simulink model "combinedTxRx"  (R2018a)
settings: Solver=FixedStepDiscrete  StartTime=0.0  StopTime=10.0  RelTol=1e-3
InitFcn:
  | modelSettings
values from neighbouring files (symbols this model uses):
  RadioSampleRate = 1e6    (= 1000000)    [modelSettings.m]
libraries: RxTxFixedPointLibrary x2, dspsigops x2, commsource2 x1
settings Model: Creator=tcollins  LastModifiedBy=fpgaws
settings OptimizationCC: BlockReduction=off  ConditionallyExecuteInputs=off  DefaultParameterBehavior=Inlined
settings DebuggingCC: AlgebraicLoopMsg=error  SingleTaskRateTransMsg=error  ParameterPrecisionLossMsg=none
settings HardwareCC: ProdBitPerPointer=32  ProdBitPerSizeT=32  ProdBitPerPtrDiffT=32  ProdLargestAtomicFloat=None  ProdIntDivRoundTo=Undefined  ProdEndianess=Unspecified  ProdWordSize=32  ProdHWDeviceType=ASIC/FPGA->ASIC/FPGA  ProdEqTarget=off
settings CodeAppCC: StateflowObjectComments=on

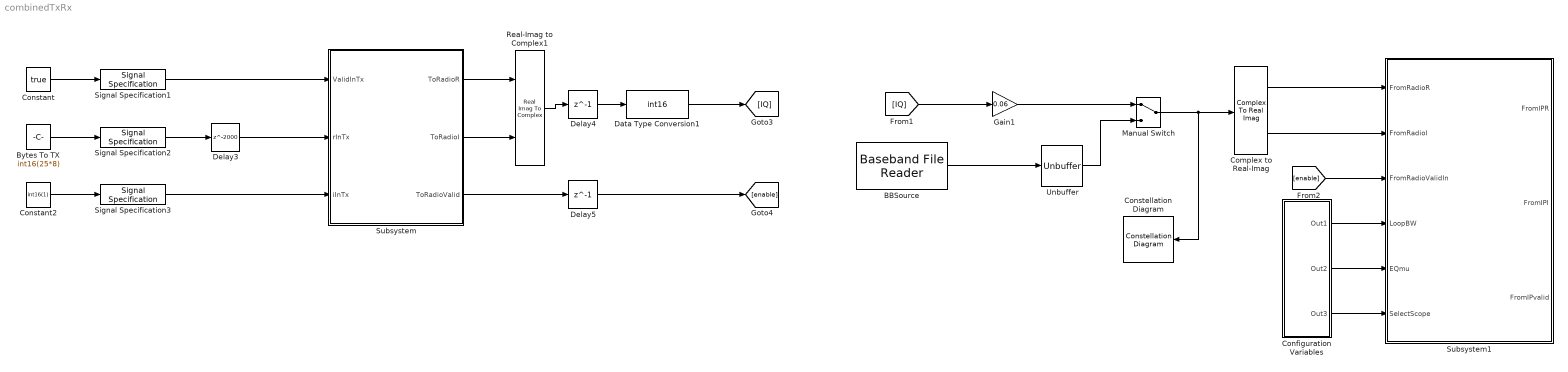
== system combinedTxRx ==
  BBSource : commsource2/Baseband File Reader  Filename=PlutoCaptureQPSK.bb  InheritSampleTimeFromFile=off  SampleTime=100000/(RadioSampleRate)  SamplesPerFrame=100000  CyclicRepetition=off  FileEndOutputPort=off  SimulateUsing=Interpreted execution
      settings: SourceProductName=Communications System Toolbox  SourceProductBaseCode=CM
  Bytes To TX : Constant  Value=int16(25*8)  SampleTime=-1
  Complex to Real-Imag : ComplexToRealImag
  Configuration Variables : Subsystem
  Constant : Constant  Value=true  SampleTime=-1
  Constant2 : Constant  Value=int16(1)  SampleTime=-1
  Constellation Diagram : ConstellationDiagram
  Data Type Conversion1 : DataTypeConversion  OutDataTypeStr=int16  ConvertRealWorld=Stored Integer (SI)
  Delay3 : Delay  DelayLength=2000
  Delay4 : Delay  DelayLength=1
  Delay5 : Delay  DelayLength=1
  Gain1 : Gain  Gain=0.06  OutDataTypeStr=int16
  Manual Switch : ManualSwitch
  Real-Imag to Complex1 : RealImagToComplex
  Signal Specification1 : SignalSpecification  OutDataTypeStr=boolean  SampleTime=1/RadioSampleRate
  Signal Specification2 : SignalSpecification  OutDataTypeStr=int16  SampleTime=1/RadioSampleRate
  Signal Specification3 : SignalSpecification  OutDataTypeStr=int16  SampleTime=1/RadioSampleRate
  Subsystem : Subsystem
  Subsystem1 : Subsystem
  Unbuffer : Unbuffer
  wires:
  Bytes To TX/1 -> Signal Specification2/1
  Constant2/1 -> Signal Specification3/1
  Constant/1 -> Signal Specification1/1
  BBSource/1 -> Unbuffer/1
  Signal Specification2/1 -> Delay3/1
  [IQ] -> Gain1/1
  Gain1/1 -> Manual Switch/1
  Unbuffer/1 -> Manual Switch/2
  Signal Specification1/1 -> Subsystem/1(ValidInTx)
  Delay3/1 -> Subsystem/2(rInTx)
  Signal Specification3/1 -> Subsystem/3(iInTx)
  Real-Imag to Complex1/1 -> Delay4/1
  Delay5/1 -> [enable]
  Data Type Conversion1/1 -> [IQ]
  Delay4/1 -> Data Type Conversion1/1
  Subsystem/3(ToRadioValid) -> Delay5/1
  Subsystem/1(ToRadioR) -> Real-Imag to Complex1/1
  Subsystem/2(ToRadioI) -> Real-Imag to Complex1/2
  Configuration Variables/1(Out1) -> Subsystem1/4(LoopBW)
  Configuration Variables/2(Out2) -> Subsystem1/5(EQmu)
  Configuration Variables/3(Out3) -> Subsystem1/6(SelectScope)
  [enable] -> Subsystem1/3(FromRadioValidIn)
  Complex to Real-Imag/2 -> Subsystem1/2(FromRadioI)
  Complex to Real-Imag/1 -> Subsystem1/1(FromRadioR)
  Manual Switch/1 -> Constellation Diagram/1, Complex to Real-Imag/1

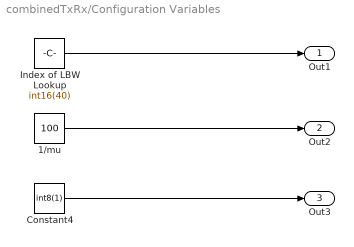
== system combinedTxRx/Configuration Variables ==
  1/mu : Constant  Value=100  OutDataTypeStr=int16  SampleTime=-1
  Constant4 : Constant  Value=int8(1)  SampleTime=1/RadioSampleRate
  Index of LBW Lookup : Constant  Value=int16(40)  SampleTime=1/RadioSampleRate
  Out1 : Outport
  Out2 : Outport  Port=2
  Out3 : Outport  Port=3
  wires:
  1/mu/1 -> Out2/1
  Index of LBW Lookup/1 -> Out1/1
  Constant4/1 -> Out3/1

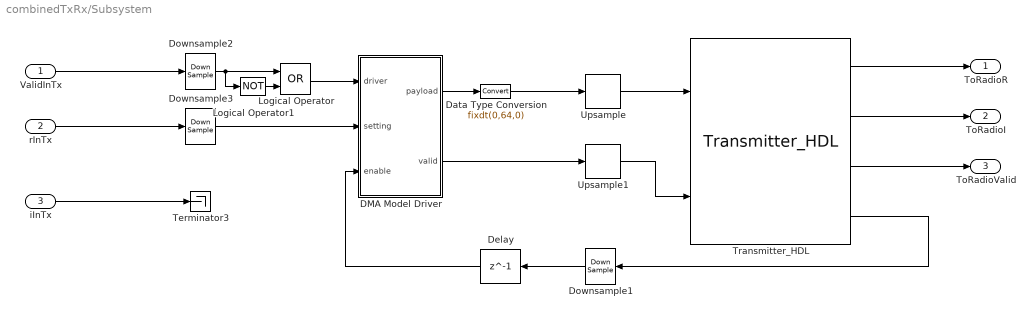
== system combinedTxRx/Subsystem ==
  ValidInTx : Inport
  rInTx : Inport  Port=2
  iInTx : Inport  Port=3
  DMA Model Driver : MATLAB Function  TreatAsAtomicUnit=on
  Data Type Conversion : DataTypeConversion  OutDataTypeStr=fixdt(0,64,0)
  Delay : Delay  DelayLength=1
  Downsample1 : DownSample  N=4  RateOptions=Allow multirate processing
  Downsample2 : DownSample  N=4  RateOptions=Allow multirate processing
  Downsample3 : DownSample  N=4  RateOptions=Allow multirate processing
  Logical Operator : Logic  Operator=OR  AllPortsSameDT=off  OutDataTypeStr=boolean
  Logical Operator1 : Logic  Operator=NOT  AllPortsSameDT=off  OutDataTypeStr=boolean
  Terminator3 : Terminator
  Transmitter_HDL : RxTxFixedPointLibrary/Transmitter_HDL  SystemSampleTime=-1
  Upsample : dspsigops/Upsample  N=4  phase=0  RateOptions=Allow multirate processing  ic=0  mode=Unused parameter value
  Upsample1 : dspsigops/Upsample  N=4  phase=0  RateOptions=Allow multirate processing  ic=0  mode=Unused parameter value
  ToRadioR : Outport
  ToRadioI : Outport  Port=2
  ToRadioValid : Outport  Port=3
  wires:
  Upsample/1 -> Transmitter_HDL/1
  Upsample1/1 -> Transmitter_HDL/2
  Transmitter_HDL/2 -> ToRadioI/1
  Downsample3/1 -> DMA Model Driver/2(setting)
  Logical Operator/1 -> DMA Model Driver/1(driver)
  Downsample2/1 -> Logical Operator/1, Logical Operator1/1
  iInTx/1 -> Terminator3/1
  Transmitter_HDL/4 -> Downsample1/1
  rInTx/1 -> Downsample3/1
  Data Type Conversion/1 -> Upsample/1
  DMA Model Driver/2(valid) -> Upsample1/1
  Transmitter_HDL/3 -> ToRadioValid/1
  Logical Operator1/1 -> Logical Operator/2
  DMA Model Driver/1(payload) -> Data Type Conversion/1
  Transmitter_HDL/1 -> ToRadioR/1
  Downsample1/1 -> Delay/1
  ValidInTx/1 -> Downsample2/1
  Delay/1 -> DMA Model Driver/3(enable)

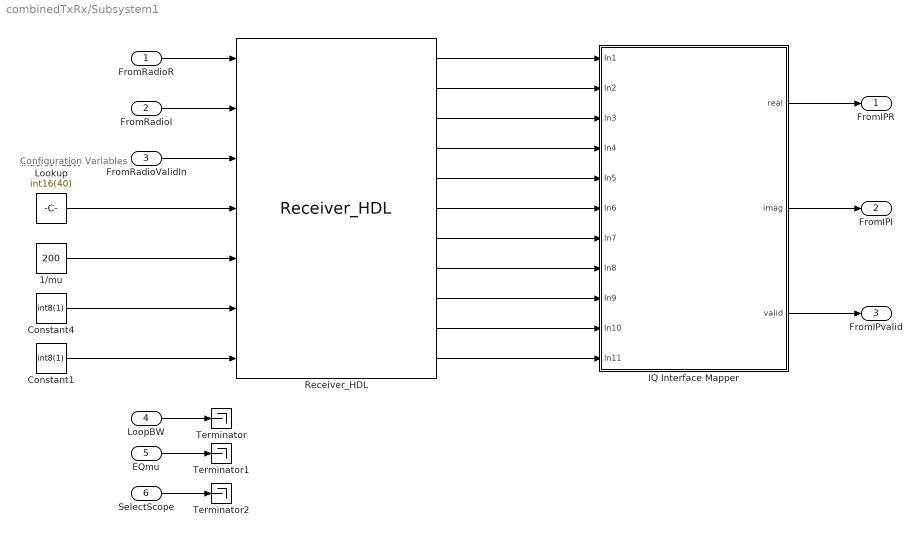
== system combinedTxRx/Subsystem1 ==
  note: Configuration
      | Variables
  FromRadioR : Inport  PortDimensions=1
  FromRadioI : Inport  Port=2  PortDimensions=1
  FromRadioValidIn : Inport  Port=3
  LoopBW : Inport  Port=4
  EQmu : Inport  Port=5
  SelectScope : Inport  Port=6
  1/mu : Constant  Value=200  OutDataTypeStr=int16  SampleTime=-1
  Constant1 : Constant  Value=int8(1)  SampleTime=1/RadioSampleRate
  Constant4 : Constant  Value=int8(1)  SampleTime=1/RadioSampleRate
  IQ Interface Mapper : Subsystem
  Index of LBW Lookup : Constant  Value=int16(40)  SampleTime=1/RadioSampleRate
  Receiver_HDL : RxTxFixedPointLibrary/Receiver_HDL  SystemSampleTime=-1
  Terminator : Terminator
  Terminator1 : Terminator
  Terminator2 : Terminator
  FromIPR : Outport
  FromIPI : Outport  Port=2
  FromIPvalid : Outport  Port=3
  wires:
  SelectScope/1 -> Terminator2/1
  LoopBW/1 -> Terminator/1
  IQ Interface Mapper/3(valid) -> FromIPvalid/1
  IQ Interface Mapper/2(imag) -> FromIPI/1
  FromRadioR/1 -> Receiver_HDL/1
  Constant4/1 -> Receiver_HDL/6
  Receiver_HDL/1 -> IQ Interface Mapper/1(In1)
  EQmu/1 -> Terminator1/1
  Constant1/1 -> Receiver_HDL/7
  FromRadioValidIn/1 -> Receiver_HDL/3
  IQ Interface Mapper/1(real) -> FromIPR/1
  1/mu/1 -> Receiver_HDL/5
  FromRadioI/1 -> Receiver_HDL/2
  Index of LBW Lookup/1 -> Receiver_HDL/4
  Receiver_HDL/2 -> IQ Interface Mapper/2(In2)
  Receiver_HDL/3 -> IQ Interface Mapper/3(In3)
  Receiver_HDL/4 -> IQ Interface Mapper/4(In4)
  Receiver_HDL/5 -> IQ Interface Mapper/5(In5)
  Receiver_HDL/6 -> IQ Interface Mapper/6(In6)
  Receiver_HDL/7 -> IQ Interface Mapper/7(In7)
  Receiver_HDL/8 -> IQ Interface Mapper/8(In8)
  Receiver_HDL/9 -> IQ Interface Mapper/9(In9)
  Receiver_HDL/10 -> IQ Interface Mapper/10(In10)
  Receiver_HDL/11 -> IQ Interface Mapper/11(In11)

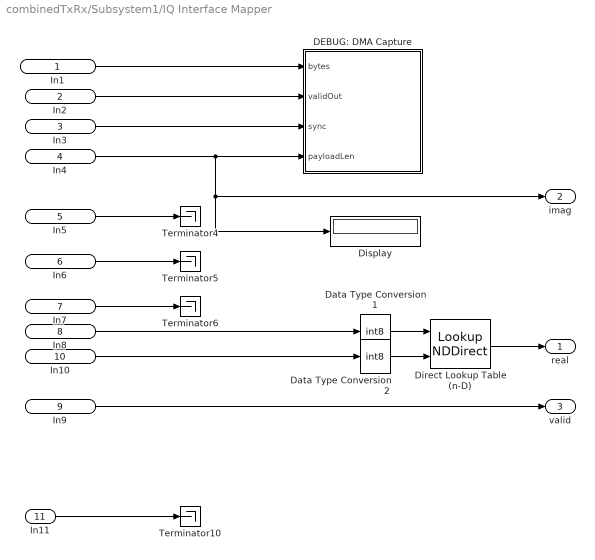
== system combinedTxRx/Subsystem1/IQ Interface Mapper ==
  In1 : Inport
  In2 : Inport  Port=2
  In3 : Inport  Port=3
  In4 : Inport  Port=4
  In5 : Inport  Port=5
  In6 : Inport  Port=6
  In7 : Inport  Port=7
  In8 : Inport  Port=8
  In9 : Inport  Port=9
  In10 : Inport  Port=10
  In11 : Inport  Port=11
  DEBUG: DMA Capture : MATLAB Function  TreatAsAtomicUnit=on
  Data Type Conversion1 : DataTypeConversion  OutDataTypeStr=int8
  Data Type Conversion2 : DataTypeConversion  OutDataTypeStr=int8
  Direct Lookup Table (n-D) : LookupNDDirect  Table=[1 2; 3 4]  DiagnosticForOutOfRangeInput=Error  TableDataTypeStr=int16
  Display : Display
  Terminator{4..6,10} (4 alike) : Terminator
  real : Outport
  imag : Outport  Port=2
  valid : Outport  Port=3
  wires:
  Data Type Conversion1/1 -> Direct Lookup Table (n-D)/1
  Data Type Conversion2/1 -> Direct Lookup Table (n-D)/2
  Direct Lookup Table (n-D)/1 -> real/1
  In1/1 -> DEBUG: DMA Capture/1(bytes)
  In2/1 -> DEBUG: DMA Capture/2(validOut)
  In3/1 -> DEBUG: DMA Capture/3(sync)
  In4/1 -> imag/1, Display/1, DEBUG: DMA Capture/4(payloadLen)
  In5/1 -> Terminator4/1
  In6/1 -> Terminator5/1
  In7/1 -> Terminator6/1
  In8/1 -> Data Type Conversion1/1
  In9/1 -> valid/1
  In10/1 -> Data Type Conversion2/1
  In11/1 -> Terminator10/1

== matlab function combinedTxRx/Subsystem/DMA Model Driver ==
  data: driver input; setting input; payload output; valid output boolean; enable input
function [payload,valid] = fcn(driver, setting, enable)
%#codegen

persistent indx mode pSize

if isempty(indx)
    pSize = fi(200,0,64,0); % Size in bytes (Must be multiple of 32 bits) cannot exceed uint16 max
    indx = pSize;
    mode = int8(0);
end


if enable && driver
    valid = true;
    switch mode
        case int8(0) % Fresh packet start
            if setting>0
                pSize = fi(setting,0,64,0);
                payload = fi(setting,0,64,0);%Upper bits
                mode = int8(1);
                indx = fi(0,0,64,0);
                %fprintf('(TX) Sending new packet with length: %u\n',uint64(pSize));
            else
                valid = false;
                payload = fi(0,0,64,0);
            end
        otherwise
            indx = fi(indx + fi(8,0,64,0),0,64,0);
            if indx == fi(8,0,64,0)
               payload = fi(0,0,64,0);
               payload = bitset(payload,1,1);
%                 payload = fi(uint64(12297829382473034410),0,64,0);%sum(2.^[0:2:14])); % Alternating ones and zeros
            elseif indx == pSize
                payload = fi(uint64(18446744073709551615),0,64,0); % All ones
%                  payload = fi(uint64(12297829382473034410),0,64,0);%sum(2.^[0:2:14])); % Alternating ones and zeros
          else
                %payload = fi(uint64(randi([0 12297829382473034410])),0,64,0);%sum(2.^[0:2:14])); % Alternating ones and zeros
                payload = fi(uint64(12297829382473034410),0,64,0);%sum(2.^[0:2:14])); % Alternating ones and zeros
            end
            if indx == pSize % reached end of frame
                mode = int8(0);
            end
    end
else
    valid = false;
    payload = fi(0,0,64,0);
end

== matlab function combinedTxRx/Subsystem1/IQ Interface Mapper/DEBUG: DMA Capture ==
  data: bytes input; validOut input; sync input; payloadLen input
function fcn(bytes, validOut, sync, payloadLen)

persistent frameBuffer byteCounter fullPayloadBits

bitsInPack = 64;

if isempty(frameBuffer)
    maxFrameBits = (2^16)*8;
    frameBuffer = false(maxFrameBits,1);
    byteCounter = 0;
    fullPayloadBits = uint16(0);
end

if validOut
    if sync
        byteCounter = bitsInPack;
        frameBuffer(1:byteCounter) = bitget(bytes,1:bitsInPack);
        fullPayloadBits = uint16(payloadLen*8);
        
    elseif byteCounter<fullPayloadBits
        frameBuffer(byteCounter+1:byteCounter+bitsInPack) = bitget(bytes,1:bitsInPack);
        byteCounter = byteCounter + bitsInPack;
    else
        if bytes>0
            disp('CRC Error (Outside)');
        else
            disp('Frame passed CRC (Outside)');
        end
    end
end
